simulink model "ScpAp_L1SpeedMonitor"  (R2025b)
settings: Solver=FixedStepDiscrete  StartTime=0.0  StopTime=10.0  FixedStep=0.01  RelTol=1e-3
model workspace (MAT data in the model file):
  Accel_Max = Simulink.Parameter
  Accel_Max.Value = 32.767
  Accel_Max.Complexity = 'real'
  Accel_Max.Dimensions = [1 1]
  Accel_Max.DataType = 'double'
  Alpha_Accel_IMU = Simulink.Parameter
  Alpha_Accel_IMU.Value = 0.15
  Alpha_Accel_IMU.Complexity = 'real'
  Alpha_Accel_IMU.Dimensions = [1 1]
  Alpha_Accel_IMU.DataType = 'double'
  Alpha_Motor = Simulink.Parameter
  Alpha_Motor.Value = 0.45
  Alpha_Motor.Complexity = 'real'
  Alpha_Motor.Dimensions = [1 1]
  Alpha_Motor.DataType = 'double'
  Alpha_WSS = Simulink.Parameter
  Alpha_WSS.Value = 0.35
  Alpha_WSS.Complexity = 'real'
  Alpha_WSS.Dimensions = [1 1]
  Alpha_WSS.DataType = 'double'
  Motor_Spd_Max = Simulink.Parameter
  Motor_Spd_Max.Value = 1023
  Motor_Spd_Max.Complexity = 'real'
  Motor_Spd_Max.Dimensions = [1 1]
  Motor_Spd_Max.DataType = 'uint16'
  Motor_Spd_Min = Simulink.Parameter
  Motor_Spd_Min.Value = 0
  Motor_Spd_Min.Complexity = 'real'
  Motor_Spd_Min.Dimensions = [1 1]
  Motor_Spd_Min.DataType = 'uint16'
  WhlSpd_Max = Simulink.Parameter
  WhlSpd_Max.Value = 32
  WhlSpd_Max.Complexity = 'real'
  WhlSpd_Max.Dimensions = [1 1]
  WhlSpd_Max.DataType = 'uint16'
  WhlSpd_Min = Simulink.Parameter
  WhlSpd_Min.Value = 0
  WhlSpd_Min.Complexity = 'real'
  WhlSpd_Min.Dimensions = [1 1]
  WhlSpd_Min.DataType = 'uint16'
undefined symbols (not defined in the file): IMU_Stuck_Delta, Motor_Stuck_Delta, Stuck_Th_Cyc, Wheel_Spd_Th, Whl_Stuck_Delta, WSS_Avg_Spd
settings Model: DataDictionary=EgasPOC.sldd  Creator=IAST283  LastModifiedBy=IAST283
settings DataIOCC: SaveFormat=StructureWithTime
settings OptimizationCC: DefaultParameterBehavior=Inlined  EnhancedBackFolding=on  PassReuseOutputArgsAs=Individual arguments  ZeroExternalMemoryAtStartup=off  ZeroInternalMemoryAtStartup=off  OptimizeBlockOrder=speed  DifferentSizesBufferReuse=on  OptimizationCustomize=off  EfficientTunableParamExpr=on
settings DebuggingCC: ParameterPrecisionLossMsg=none  ParameterTunabilityLossMsg=error
settings SFSimCC: MATLABDynamicMemAlloc=off
settings RTWCC: SystemTargetFile=autosar.tlc  GenCodeOnly=on  TemplateMakefile=ert_default_tmf  GenerateReport=on  DataTypeReplacement=CDataTypesFixedWidth  Description=AUTOSAR
settings CodeAppCC: ForceParamTrailComments=on  IgnoreCustomStorageClasses=off  OperatorAnnotations=on  SimulinkDataObjDesc=on  SFDataObjDesc=on  InsertBlockDesc=on
settings STFCustomTargetCC: SystemTargetFile=autosar.tlc  TargetLangStandard=C99 (ISO)  MultiwordLength=256.0  ParMdlRefBuildCompliant=on  CompOptLevelCompliant=on  ConcurrentExecutionCompliant=off  IncludeMdlTerminateFcn=off  CombineOutputUpdateFcns=on  SuppressErrorStatus=on  ERTCustomFileBanners=on  SupportNonFinite=off  SupportComplex=off  SupportContinuousTime=off  SupportNonInlinedSFcns=off  RemoveResetFunc=on  MATLABClassNameForMDSCustomization=Simulink.SoftwareTarget.ERTCustomization  AutosarCompliant=on  GRTInterface=off  UseToolchainInfoCompliant=on  LookupTableObjectStructAxisOrder=2,1,3,4,...  LUTObjectStructOrderEvenSpacing=Size,Table,Breakpoints  AutosarMatrixIOAsArray=off  DisableAUTOSARRoutinesHostLibrary=off  AutosarCompilerAbstraction=off  AutosarSchemaVersion=R23-11  AutosarMaxShortNameLength=128.0
settings ERTTargetCC: ERTCustomFileTemplate=example_file_process.tlc  BooleanTrueId=TRUE  BooleanFalseId=FALSE  TargetLangStandard=C99 (ISO)  ConcurrentExecutionCompliant=off  IncludeMdlTerminateFcn=off  SuppressErrorStatus=on  SupportNonFinite=off  SupportComplex=off  ModelStepFunctionPrototypeControlCompliant=off  CPPClassGenCompliant=off  AutosarCompliant=on  LookupTableObjectStructAxisOrder=2,1,3,4,...  LUTObjectStructOrderEvenSpacing=Size,Table,Breakpoints

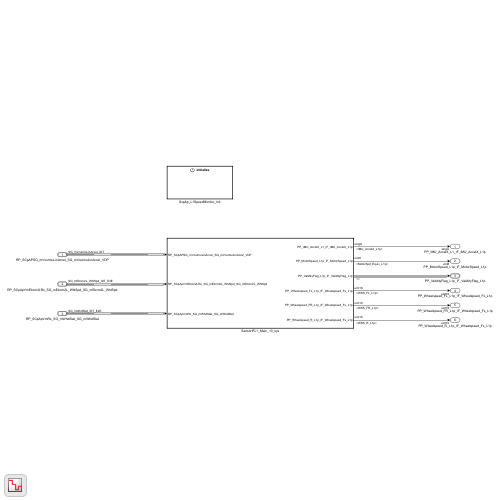
[thumbnail: Simulink's stored preview of the top-level diagram]
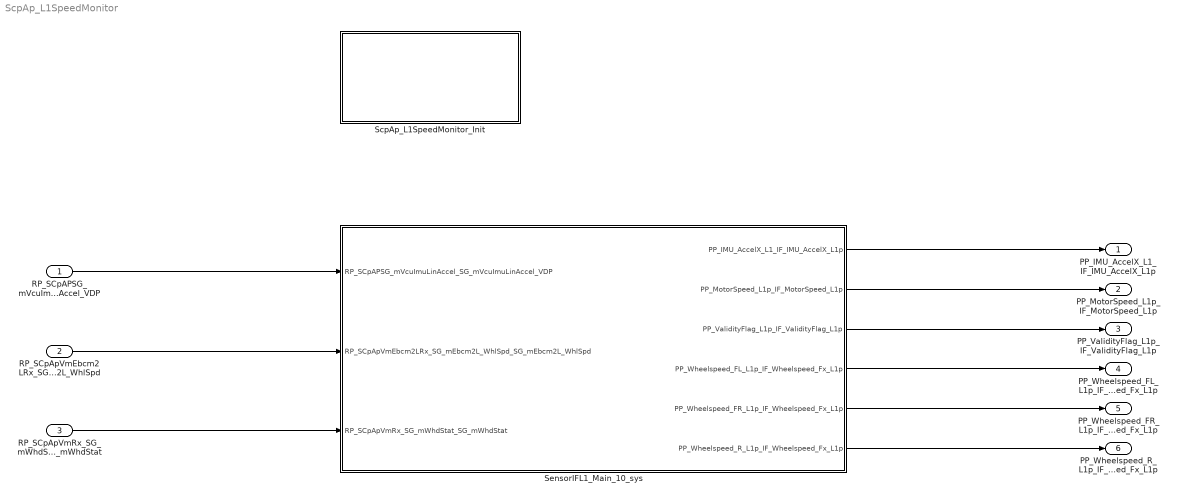
== system ScpAp_L1SpeedMonitor ==
  RP_SCpAPSG_mVcuImuLinAccel_SG_mVcuImuLinAccel_VDP : Inport  OutDataTypeStr=Bus: SG_mVcuImuLinAccel_IDT  PortDimensions=1  BusOutputAsStruct=on
  RP_SCpApVmEbcm2LRx_SG_mEbcm2L_WhlSpd_SG_mEbcm2L_WhlSpd : Inport  Port=2  OutDataTypeStr=Bus: SG_mEbcm2L_WhlSpd_IDT_E2E  PortDimensions=1  BusOutputAsStruct=on
  RP_SCpApVmRx_SG_mWhdStat_SG_mWhdStat : Inport  Port=3  OutDataTypeStr=Bus: SG_mWhdStat_IDT_E2E  PortDimensions=1  BusOutputAsStruct=on
  ScpAp_L1SpeedMonitor_Init : Subsystem
  SensorIFL1_Main_10_sys : Subsystem  TreatAsAtomicUnit=on  SystemSampleTime=0.01
  PP_IMU_AccelX_L1_IF_IMU_AccelX_L1p : Outport  OutDataTypeStr=single  PortDimensions=1
  PP_MotorSpeed_L1p_IF_MotorSpeed_L1p : Outport  Port=2  OutDataTypeStr=uint8  PortDimensions=1
  PP_ValidityFlag_L1p_IF_ValidityFlag_L1p : Outport  Port=3  OutDataTypeStr=Bus: IF_ValidityFlag_L1p_IDT  PortDimensions=1  BusOutputAsStruct=on
  PP_Wheelspeed_FL_L1p_IF_Wheelspeed_Fx_L1p : Outport  Port=4  OutDataTypeStr=uint16  PortDimensions=1
  PP_Wheelspeed_FR_L1p_IF_Wheelspeed_Fx_L1p : Outport  Port=5  OutDataTypeStr=uint16  PortDimensions=1
  PP_Wheelspeed_R_L1p_IF_Wheelspeed_Fx_L1p : Outport  Port=6  OutDataTypeStr=uint16  PortDimensions=1
  wires:
  RP_SCpAPSG_mVcuImuLinAccel_SG_mVcuImuLinAccel_VDP/1 -> SensorIFL1_Main_10_sys/1(RP_SCpAPSG_mVcuImuLinAccel_SG_mVcuImuLinAccel_VDP)
  RP_SCpApVmEbcm2LRx_SG_mEbcm2L_WhlSpd_SG_mEbcm2L_WhlSpd/1 -> SensorIFL1_Main_10_sys/2(RP_SCpApVmEbcm2LRx_SG_mEbcm2L_WhlSpd_SG_mEbcm2L_WhlSpd)
  RP_SCpApVmRx_SG_mWhdStat_SG_mWhdStat/1 -> SensorIFL1_Main_10_sys/3(RP_SCpApVmRx_SG_mWhdStat_SG_mWhdStat)
  SensorIFL1_Main_10_sys/1(PP_IMU_AccelX_L1_IF_IMU_AccelX_L1p) -> PP_IMU_AccelX_L1_IF_IMU_AccelX_L1p/1
  SensorIFL1_Main_10_sys/2(PP_MotorSpeed_L1p_IF_MotorSpeed_L1p) -> PP_MotorSpeed_L1p_IF_MotorSpeed_L1p/1
  SensorIFL1_Main_10_sys/3(PP_ValidityFlag_L1p_IF_ValidityFlag_L1p) -> PP_ValidityFlag_L1p_IF_ValidityFlag_L1p/1
  SensorIFL1_Main_10_sys/4(PP_Wheelspeed_FL_L1p_IF_Wheelspeed_Fx_L1p) -> PP_Wheelspeed_FL_L1p_IF_Wheelspeed_Fx_L1p/1
  SensorIFL1_Main_10_sys/5(PP_Wheelspeed_FR_L1p_IF_Wheelspeed_Fx_L1p) -> PP_Wheelspeed_FR_L1p_IF_Wheelspeed_Fx_L1p/1
  SensorIFL1_Main_10_sys/6(PP_Wheelspeed_R_L1p_IF_Wheelspeed_Fx_L1p) -> PP_Wheelspeed_R_L1p_IF_Wheelspeed_Fx_L1p/1

== system ScpAp_L1SpeedMonitor/ScpAp_L1SpeedMonitor_Init ==
  Event Listener : EventListener  EventName=reset

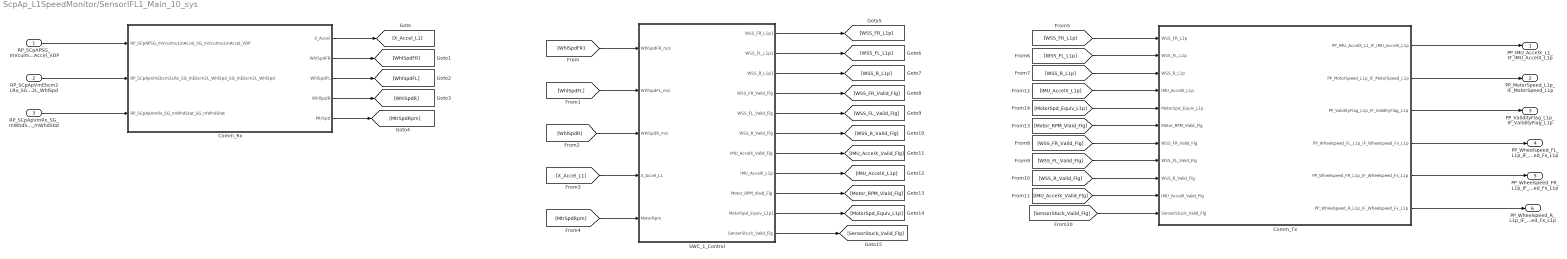
== system ScpAp_L1SpeedMonitor/SensorIFL1_Main_10_sys ==
  RP_SCpAPSG_mVcuImuLinAccel_SG_mVcuImuLinAccel_VDP : Inport
  RP_SCpApVmEbcm2LRx_SG_mEbcm2L_WhlSpd_SG_mEbcm2L_WhlSpd : Inport  Port=2
  RP_SCpApVmRx_SG_mWhdStat_SG_mWhdStat : Inport  Port=3
  Comm_Rx : Subsystem
  Comm_Tx : Subsystem
  SWC_1_Control : Subsystem  TreatAsAtomicUnit=on
  PP_IMU_AccelX_L1_IF_IMU_AccelX_L1p : Outport
  PP_MotorSpeed_L1p_IF_MotorSpeed_L1p : Outport  Port=2
  PP_ValidityFlag_L1p_IF_ValidityFlag_L1p : Outport  Port=3
  PP_Wheelspeed_FL_L1p_IF_Wheelspeed_Fx_L1p : Outport  Port=4
  PP_Wheelspeed_FR_L1p_IF_Wheelspeed_Fx_L1p : Outport  Port=5
  PP_Wheelspeed_R_L1p_IF_Wheelspeed_Fx_L1p : Outport  Port=6
  wires:
  Comm_Rx/3(WhlSpdFL) -> [WhlSpdFL]
  Comm_Rx/5(MtrSpd) -> [MtrSpdRpm]
  Comm_Rx/4(WhlSpdR) -> [WhlSpdR]
  Comm_Rx/2(WhlSpdFR) -> [WhlSpdFR]
  Comm_Rx/1(X_Accel) -> [X_Accel_L1]
  RP_SCpAPSG_mVcuImuLinAccel_SG_mVcuImuLinAccel_VDP/1 -> Comm_Rx/1(RP_SCpAPSG_mVcuImuLinAccel_SG_mVcuImuLinAccel_VDP)
  RP_SCpApVmRx_SG_mWhdStat_SG_mWhdStat/1 -> Comm_Rx/3(RP_SCpApVmRx_SG_mWhdStat_SG_mWhdStat)
  RP_SCpApVmEbcm2LRx_SG_mEbcm2L_WhlSpd_SG_mEbcm2L_WhlSpd/1 -> Comm_Rx/2(RP_SCpApVmEbcm2LRx_SG_mEbcm2L_WhlSpd_SG_mEbcm2L_WhlSpd)
  SWC_1_Control/7(IMU_AccelX_Valid_Flg) -> [IMU_AccelX_Valid_Flg]
  [WhlSpdFL] -> SWC_1_Control/2(WhlSpdFL_m/s)
  SWC_1_Control/1(WSS_FR_L1p1) -> [WSS_FR_L1p]
  SWC_1_Control/4(WSS_FR_Valid_Flg) -> [WSS_FR_Valid_Flg]
  SWC_1_Control/6(WSS_R_Valid_Flg) -> [WSS_R_Valid_Flg]
  SWC_1_Control/2(WSS_FL_L1p1) -> [WSS_FL_L1p]
  SWC_1_Control/11(SensorStuck_Valid_Flg) -> [SensorStuck_Valid_Flg]
  SWC_1_Control/9(Motor_RPM_Vlaid_Flg) -> [Motor_RPM_Vlaid_Flg]
  SWC_1_Control/10(MotorSpd_Equiv_L1p1) -> [MotorSpd_Equiv_L1p]
  SWC_1_Control/8(IMU_AccelX_L1p) -> [IMU_AccelX_L1p]
  SWC_1_Control/3(WSS_R_L1p1) -> [WSS_R_L1p]
  [MtrSpdRpm] -> SWC_1_Control/5(MotorRpm)
  [WhlSpdFR] -> SWC_1_Control/1(WhlSpdFR_m/s)
  [WhlSpdR] -> SWC_1_Control/3(WhlSpdR_m/s)
  SWC_1_Control/5(WSS_FL_Valid_Flg) -> [WSS_FL_Valid_Flg]
  [X_Accel_L1] -> SWC_1_Control/4(X_Accel_L1)
  [WSS_FR_L1p] -> Comm_Tx/1(WSS_FR_L1p)
  [WSS_FL_L1p] -> Comm_Tx/2(WSS_FL_L1p)
  [WSS_R_L1p] -> Comm_Tx/3(WSS_R_L1p)
  [IMU_AccelX_L1p] -> Comm_Tx/4(IMU_AccelX_L1p)
  [MotorSpd_Equiv_L1p] -> Comm_Tx/5(MotorSpd_Equiv_L1p)
  [Motor_RPM_Vlaid_Flg] -> Comm_Tx/6(Motor_RPM_Valid_Flg)
  [WSS_FR_Valid_Flg] -> Comm_Tx/7(WSS_FR_Valid_Flg)
  [WSS_FL_Valid_Flg] -> Comm_Tx/8(WSS_FL_Valid_Flg)
  [SensorStuck_Valid_Flg] -> Comm_Tx/11(SensorStuck_Valid_Flg)
  [IMU_AccelX_Valid_Flg] -> Comm_Tx/10(IMU_AccelX_Valid_Flg)
  [WSS_R_Valid_Flg] -> Comm_Tx/9(WSS_R_Valid_Flg)
  Comm_Tx/1(PP_IMU_AccelX_L1_IF_IMU_AccelX_L1p) -> PP_IMU_AccelX_L1_IF_IMU_AccelX_L1p/1
  Comm_Tx/2(PP_MotorSpeed_L1p_IF_MotorSpeed_L1p) -> PP_MotorSpeed_L1p_IF_MotorSpeed_L1p/1
  Comm_Tx/3(PP_ValidityFlag_L1p_IF_ValidityFlag_L1p) -> PP_ValidityFlag_L1p_IF_ValidityFlag_L1p/1
  Comm_Tx/4(PP_Wheelspeed_FL_L1p_IF_Wheelspeed_Fx_L1p) -> PP_Wheelspeed_FL_L1p_IF_Wheelspeed_Fx_L1p/1
  Comm_Tx/5(PP_Wheelspeed_FR_L1p_IF_Wheelspeed_Fx_L1p) -> PP_Wheelspeed_FR_L1p_IF_Wheelspeed_Fx_L1p/1
  Comm_Tx/6(PP_Wheelspeed_R_L1p_IF_Wheelspeed_Fx_L1p) -> PP_Wheelspeed_R_L1p_IF_Wheelspeed_Fx_L1p/1

== system ScpAp_L1SpeedMonitor/SensorIFL1_Main_10_sys/Comm_Rx ==
  RP_SCpAPSG_mVcuImuLinAccel_SG_mVcuImuLinAccel_VDP : Inport
  RP_SCpApVmEbcm2LRx_SG_mEbcm2L_WhlSpd_SG_mEbcm2L_WhlSpd : Inport  Port=2
  RP_SCpApVmRx_SG_mWhdStat_SG_mWhdStat : Inport  Port=3
  mEbcm2L_WhlSpd : Subsystem
  mVculmuLinAccel : Subsystem
  mWhdStat : Subsystem
  X_Accel : Outport
  WhlSpdFR : Outport  Port=2
  WhlSpdFL : Outport  Port=3
  WhlSpdR : Outport  Port=4
  MtrSpd : Outport  Port=5
  wires:
  mEbcm2L_WhlSpd/1(WhlSpdFR) -> WhlSpdFR/1
  mEbcm2L_WhlSpd/2(WhlSpdFL) -> WhlSpdFL/1
  mEbcm2L_WhlSpd/3(WhlSpdR) -> WhlSpdR/1
  RP_SCpApVmEbcm2LRx_SG_mEbcm2L_WhlSpd_SG_mEbcm2L_WhlSpd/1 -> mEbcm2L_WhlSpd/1(RP_SCpApVmEbcm2LRx_SG_mEbcm2L_WhlSpd_SG_mEbcm2L_WhlSpd)
  RP_SCpAPSG_mVcuImuLinAccel_SG_mVcuImuLinAccel_VDP/1 -> mVculmuLinAccel/1(RP_SCpAPSG_mVcuImuLinAccel_SG_mVcuImuLinAccel_VDP)
  RP_SCpApVmRx_SG_mWhdStat_SG_mWhdStat/1 -> mWhdStat/1(RP_SCpApVmRx_SG_mWhdStat_SG_mWhdStat)
  mWhdStat/1(MtrSpd) -> MtrSpd/1
  mVculmuLinAccel/1(X_Accel) -> X_Accel/1

== system ScpAp_L1SpeedMonitor/SensorIFL1_Main_10_sys/Comm_Tx ==
  WSS_FR_L1p : Inport
  WSS_FL_L1p : Inport  Port=2
  WSS_R_L1p : Inport  Port=3
  IMU_AccelX_L1p : Inport  Port=4
  MotorSpd_Equiv_L1p : Inport  Port=5
  Motor_RPM_Valid_Flg : Inport  Port=6
  WSS_FR_Valid_Flg : Inport  Port=7
  WSS_FL_Valid_Flg : Inport  Port=8
  WSS_R_Valid_Flg : Inport  Port=9
  IMU_AccelX_Valid_Flg : Inport  Port=10
  SensorStuck_Valid_Flg : Inport  Port=11
  Bus Creator : BusCreator  Inputs=6
  PP_IMU_AccelX_L1_IF_IMU_AccelX_L1p : Outport
  PP_MotorSpeed_L1p_IF_MotorSpeed_L1p : Outport  Port=2
  PP_ValidityFlag_L1p_IF_ValidityFlag_L1p : Outport  Port=3
  PP_Wheelspeed_FL_L1p_IF_Wheelspeed_Fx_L1p : Outport  Port=4
  PP_Wheelspeed_FR_L1p_IF_Wheelspeed_Fx_L1p : Outport  Port=5
  PP_Wheelspeed_R_L1p_IF_Wheelspeed_Fx_L1p : Outport  Port=6
  wires:
  WSS_FL_L1p/1 -> PP_Wheelspeed_FL_L1p_IF_Wheelspeed_Fx_L1p/1  "WSS_FL_L1p"
  WSS_FR_L1p/1 -> PP_Wheelspeed_FR_L1p_IF_Wheelspeed_Fx_L1p/1  "WSS_FR_L1p"
  WSS_R_L1p/1 -> PP_Wheelspeed_R_L1p_IF_Wheelspeed_Fx_L1p/1  "WSS_R_L1p"
  IMU_AccelX_L1p/1 -> PP_IMU_AccelX_L1_IF_IMU_AccelX_L1p/1  "IMU_AccelX_L1p"
  MotorSpd_Equiv_L1p/1 -> PP_MotorSpeed_L1p_IF_MotorSpeed_L1p/1  "MotorSpd_Equiv_L1p"
  Bus Creator/1 -> PP_ValidityFlag_L1p_IF_ValidityFlag_L1p/1
  Motor_RPM_Valid_Flg/1 -> Bus Creator/1
  WSS_FR_Valid_Flg/1 -> Bus Creator/2
  WSS_FL_Valid_Flg/1 -> Bus Creator/3
  WSS_R_Valid_Flg/1 -> Bus Creator/4
  IMU_AccelX_Valid_Flg/1 -> Bus Creator/5
  SensorStuck_Valid_Flg/1 -> Bus Creator/6

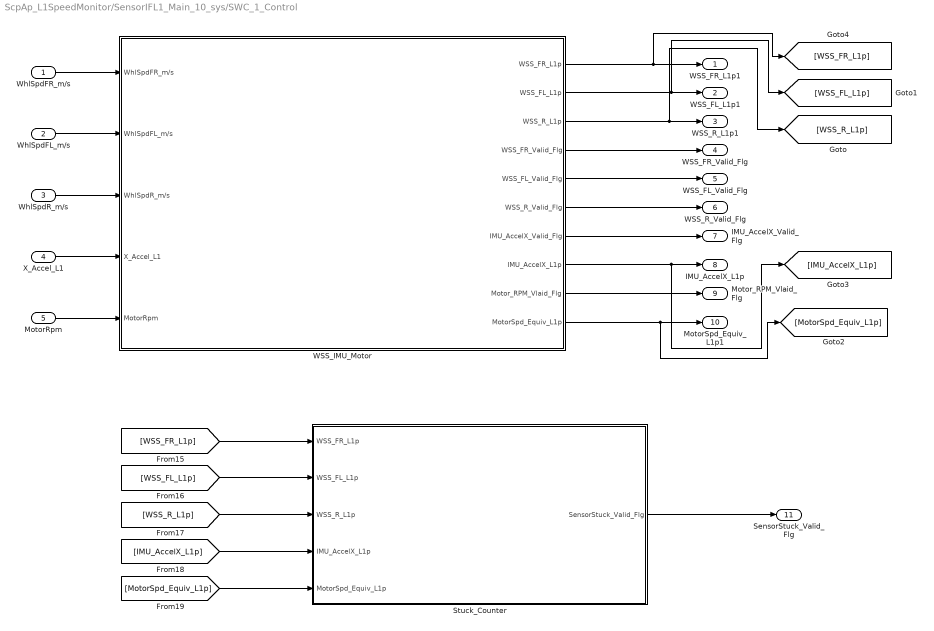
== system ScpAp_L1SpeedMonitor/SensorIFL1_Main_10_sys/SWC_1_Control ==
  WhlSpdFR_m/s : Inport
  WhlSpdFL_m/s : Inport  Port=2
  WhlSpdR_m/s : Inport  Port=3
  X_Accel_L1 : Inport  Port=4
  MotorRpm : Inport  Port=5
  Stuck_Counter : Subsystem  TreatAsAtomicUnit=on
  WSS_IMU_Motor : Subsystem  TreatAsAtomicUnit=on
  WSS_FR_L1p1 : Outport
  WSS_FL_L1p1 : Outport  Port=2
  WSS_R_L1p1 : Outport  Port=3
  WSS_FR_Valid_Flg : Outport  Port=4
  WSS_FL_Valid_Flg : Outport  Port=5
  WSS_R_Valid_Flg : Outport  Port=6
  IMU_AccelX_Valid_Flg : Outport  Port=7
  IMU_AccelX_L1p : Outport  Port=8
  Motor_RPM_Vlaid_Flg : Outport  Port=9
  MotorSpd_Equiv_L1p1 : Outport  Port=10
  SensorStuck_Valid_Flg : Outport  Port=11
  wires:
  WSS_IMU_Motor/6(WSS_R_Valid_Flg) -> WSS_R_Valid_Flg/1
  WSS_IMU_Motor/1(WSS_FR_L1p) -> WSS_FR_L1p1/1, [WSS_FR_L1p]
  WSS_IMU_Motor/9(Motor_RPM_Vlaid_Flg) -> Motor_RPM_Vlaid_Flg/1
  WSS_IMU_Motor/2(WSS_FL_L1p) -> [WSS_FL_L1p], WSS_FL_L1p1/1
  WSS_IMU_Motor/4(WSS_FR_Valid_Flg) -> WSS_FR_Valid_Flg/1
  WSS_IMU_Motor/8(IMU_AccelX_L1p) -> [IMU_AccelX_L1p], IMU_AccelX_L1p/1
  WSS_IMU_Motor/7(IMU_AccelX_Valid_Flg) -> IMU_AccelX_Valid_Flg/1
  X_Accel_L1/1 -> WSS_IMU_Motor/4(X_Accel_L1)
  Stuck_Counter/1(SensorStuck_Valid_Flg) -> SensorStuck_Valid_Flg/1
  WhlSpdR_m/s/1 -> WSS_IMU_Motor/3(WhlSpdR_m/s)
  WhlSpdFR_m/s/1 -> WSS_IMU_Motor/1(WhlSpdFR_m/s)
  WSS_IMU_Motor/3(WSS_R_L1p) -> [WSS_R_L1p], WSS_R_L1p1/1
  MotorRpm/1 -> WSS_IMU_Motor/5(MotorRpm)
  WSS_IMU_Motor/10(MotorSpd_Equiv_L1p) -> [MotorSpd_Equiv_L1p], MotorSpd_Equiv_L1p1/1
  WSS_IMU_Motor/5(WSS_FL_Valid_Flg) -> WSS_FL_Valid_Flg/1
  WhlSpdFL_m/s/1 -> WSS_IMU_Motor/2(WhlSpdFL_m/s)
  [WSS_FR_L1p] -> Stuck_Counter/1(WSS_FR_L1p)
  [WSS_FL_L1p] -> Stuck_Counter/2(WSS_FL_L1p)
  [WSS_R_L1p] -> Stuck_Counter/3(WSS_R_L1p)
  [IMU_AccelX_L1p] -> Stuck_Counter/4(IMU_AccelX_L1p)
  [MotorSpd_Equiv_L1p] -> Stuck_Counter/5(MotorSpd_Equiv_L1p)

== system ScpAp_L1SpeedMonitor/SensorIFL1_Main_10_sys/Comm_Rx/mEbcm2L_WhlSpd ==
  RP_SCpApVmEbcm2LRx_SG_mEbcm2L_WhlSpd_SG_mEbcm2L_WhlSpd : Inport
  Bus Selector : BusSelector  OutputSignals=WhlSpdFR,WhlSpdFL,WhlSpdR
  WhlSpdFR : Outport
  WhlSpdFL : Outport  Port=2
  WhlSpdR : Outport  Port=3
  wires:
  RP_SCpApVmEbcm2LRx_SG_mEbcm2L_WhlSpd_SG_mEbcm2L_WhlSpd/1 -> Bus Selector/1
  Bus Selector/1 -> WhlSpdFR/1  "<WhlSpdFR>"
  Bus Selector/2 -> WhlSpdFL/1  "<WhlSpdFL>"
  Bus Selector/3 -> WhlSpdR/1  "<WhlSpdR>"

== system ScpAp_L1SpeedMonitor/SensorIFL1_Main_10_sys/Comm_Rx/mVculmuLinAccel ==
  RP_SCpAPSG_mVcuImuLinAccel_SG_mVcuImuLinAccel_VDP : Inport
  Bus Selector : BusSelector  OutputSignals=X_Accel
  X_Accel : Outport
  wires:
  RP_SCpAPSG_mVcuImuLinAccel_SG_mVcuImuLinAccel_VDP/1 -> Bus Selector/1
  Bus Selector/1 -> X_Accel/1  "<X_Accel>"

== system ScpAp_L1SpeedMonitor/SensorIFL1_Main_10_sys/Comm_Rx/mWhdStat ==
  RP_SCpApVmRx_SG_mWhdStat_SG_mWhdStat : Inport
  Bus Selector : BusSelector  OutputSignals=MtrSpd
  MtrSpd : Outport
  wires:
  RP_SCpApVmRx_SG_mWhdStat_SG_mWhdStat/1 -> Bus Selector/1
  Bus Selector/1 -> MtrSpd/1  "<MtrSpd>"

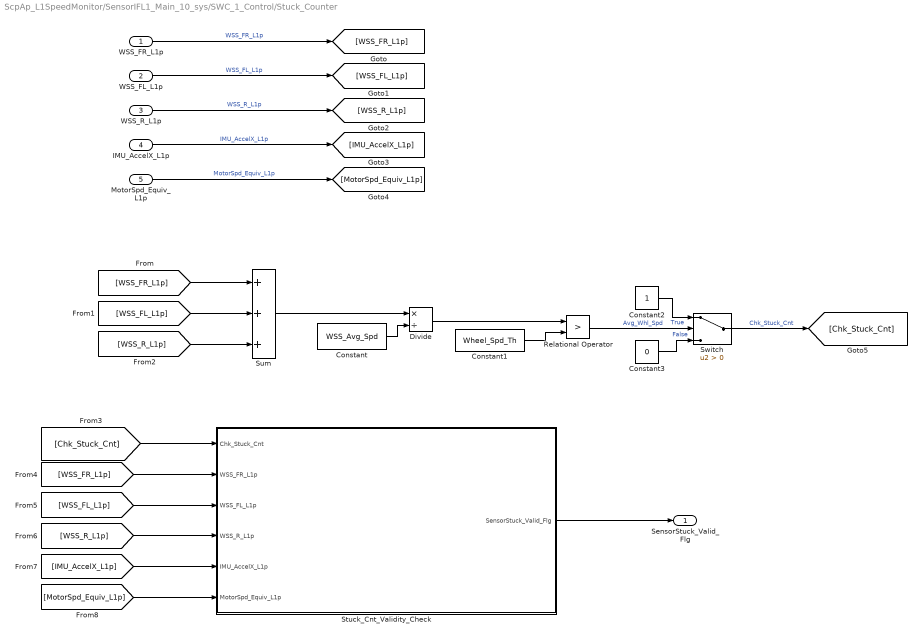
== system ScpAp_L1SpeedMonitor/SensorIFL1_Main_10_sys/SWC_1_Control/Stuck_Counter ==
  WSS_FR_L1p : Inport
  WSS_FL_L1p : Inport  Port=2
  WSS_R_L1p : Inport  Port=3
  IMU_AccelX_L1p : Inport  Port=4
  MotorSpd_Equiv_L1p : Inport  Port=5
  Constant : Constant  Value=WSS_Avg_Spd
  Constant1 : Constant  Value=Wheel_Spd_Th
  Constant2 : Constant  OutDataTypeStr=boolean
  Constant3 : Constant  Value=0  OutDataTypeStr=boolean
  Divide : Product  Inputs=*/
  Relational Operator : RelationalOperator  Operator=>  OutDataTypeStr=boolean  RndMeth=Simplest  InputSameDT=off
  Stuck_Cnt_Validity_Check : Subsystem  TreatAsAtomicUnit=on
  Sum : Sum  Inputs=+++
  Switch : Switch  Criteria=u2 > Threshold  SaturateOnIntegerOverflow=off  InputSameDT=off
  SensorStuck_Valid_Flg : Outport
  wires:
  WSS_FR_L1p/1 -> [WSS_FR_L1p]  "WSS_FR_L1p"
  WSS_FL_L1p/1 -> [WSS_FL_L1p]  "WSS_FL_L1p"
  WSS_R_L1p/1 -> [WSS_R_L1p]  "WSS_R_L1p"
  IMU_AccelX_L1p/1 -> [IMU_AccelX_L1p]  "IMU_AccelX_L1p"
  MotorSpd_Equiv_L1p/1 -> [MotorSpd_Equiv_L1p]  "MotorSpd_Equiv_L1p"
  [WSS_FR_L1p] -> Sum/1
  [WSS_FL_L1p] -> Sum/2
  [WSS_R_L1p] -> Sum/3
  Sum/1 -> Divide/1
  Constant/1 -> Divide/2
  Divide/1 -> Relational Operator/1
  Constant1/1 -> Relational Operator/2
  Relational Operator/1 -> Switch/2  "Avg_Whl_Spd"
  Constant2/1 -> Switch/1  "True"
  Constant3/1 -> Switch/3  "False"
  Switch/1 -> [Chk_Stuck_Cnt]  "Chk_Stuck_Cnt"
  [WSS_FR_L1p] -> Stuck_Cnt_Validity_Check/2(WSS_FR_L1p)
  [WSS_FL_L1p] -> Stuck_Cnt_Validity_Check/3(WSS_FL_L1p)
  [WSS_R_L1p] -> Stuck_Cnt_Validity_Check/4(WSS_R_L1p)
  [MotorSpd_Equiv_L1p] -> Stuck_Cnt_Validity_Check/6(MotorSpd_Equiv_L1p)
  [IMU_AccelX_L1p] -> Stuck_Cnt_Validity_Check/5(IMU_AccelX_L1p)
  [Chk_Stuck_Cnt] -> Stuck_Cnt_Validity_Check/1(Chk_Stuck_Cnt)
  Stuck_Cnt_Validity_Check/1(SensorStuck_Valid_Flg) -> SensorStuck_Valid_Flg/1

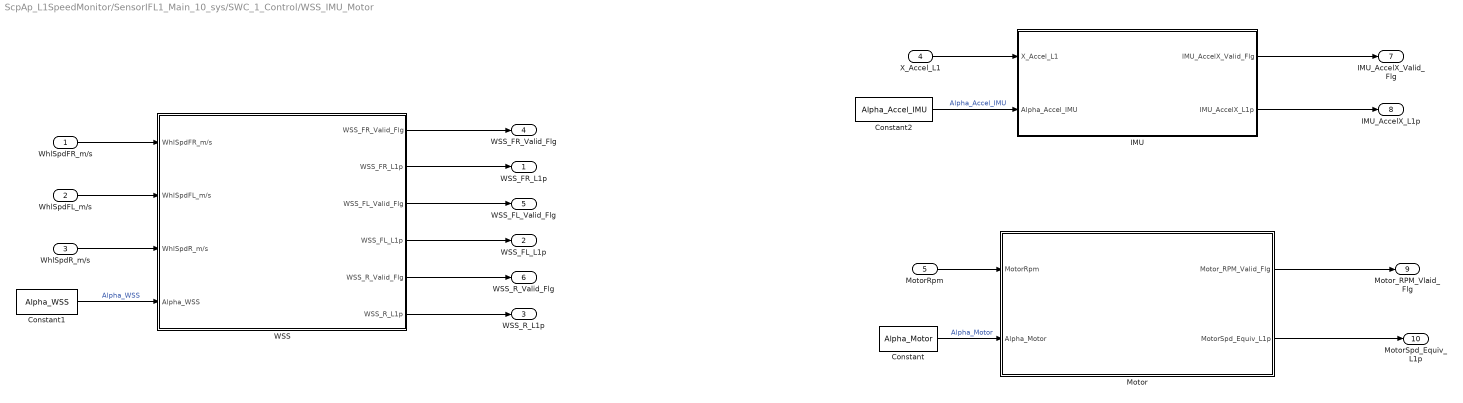
== system ScpAp_L1SpeedMonitor/SensorIFL1_Main_10_sys/SWC_1_Control/WSS_IMU_Motor ==
  WhlSpdFR_m/s : Inport
  WhlSpdFL_m/s : Inport  Port=2
  WhlSpdR_m/s : Inport  Port=3
  X_Accel_L1 : Inport  Port=4
  MotorRpm : Inport  Port=5
  Constant : Constant  Value=Alpha_Motor  OutDataTypeStr=double
  Constant1 : Constant  Value=Alpha_WSS  OutDataTypeStr=double
  Constant2 : Constant  Value=Alpha_Accel_IMU  OutDataTypeStr=double
  IMU : Subsystem  TreatAsAtomicUnit=on
  Motor : Subsystem  TreatAsAtomicUnit=on
  WSS : Subsystem  TreatAsAtomicUnit=on
  WSS_FR_L1p : Outport
  WSS_FL_L1p : Outport  Port=2
  WSS_R_L1p : Outport  Port=3
  WSS_FR_Valid_Flg : Outport  Port=4  OutDataTypeStr=boolean
  WSS_FL_Valid_Flg : Outport  Port=5
  WSS_R_Valid_Flg : Outport  Port=6
  IMU_AccelX_Valid_Flg : Outport  Port=7
  IMU_AccelX_L1p : Outport  Port=8
  Motor_RPM_Vlaid_Flg : Outport  Port=9
  MotorSpd_Equiv_L1p : Outport  Port=10
  wires:
  WSS/5(WSS_R_Valid_Flg) -> WSS_R_Valid_Flg/1
  WhlSpdR_m/s/1 -> WSS/3(WhlSpdR_m/s)
  WSS/3(WSS_FL_Valid_Flg) -> WSS_FL_Valid_Flg/1
  WSS/4(WSS_FL_L1p) -> WSS_FL_L1p/1
  WhlSpdFR_m/s/1 -> WSS/1(WhlSpdFR_m/s)
  WSS/1(WSS_FR_Valid_Flg) -> WSS_FR_Valid_Flg/1
  WSS/6(WSS_R_L1p) -> WSS_R_L1p/1
  WSS/2(WSS_FR_L1p) -> WSS_FR_L1p/1
  WhlSpdFL_m/s/1 -> WSS/2(WhlSpdFL_m/s)
  X_Accel_L1/1 -> IMU/1(X_Accel_L1)
  IMU/1(IMU_AccelX_Valid_Flg) -> IMU_AccelX_Valid_Flg/1
  IMU/2(IMU_AccelX_L1p) -> IMU_AccelX_L1p/1
  MotorRpm/1 -> Motor/1(MotorRpm)
  Motor/1(Motor_RPM_Valid_Flg) -> Motor_RPM_Vlaid_Flg/1
  Motor/2(MotorSpd_Equiv_L1p) -> MotorSpd_Equiv_L1p/1
  Constant/1 -> Motor/2(Alpha_Motor)  "Alpha_Motor"
  Constant1/1 -> WSS/4(Alpha_WSS)  "Alpha_WSS"
  Constant2/1 -> IMU/2(Alpha_Accel_IMU)  "Alpha_Accel_IMU"

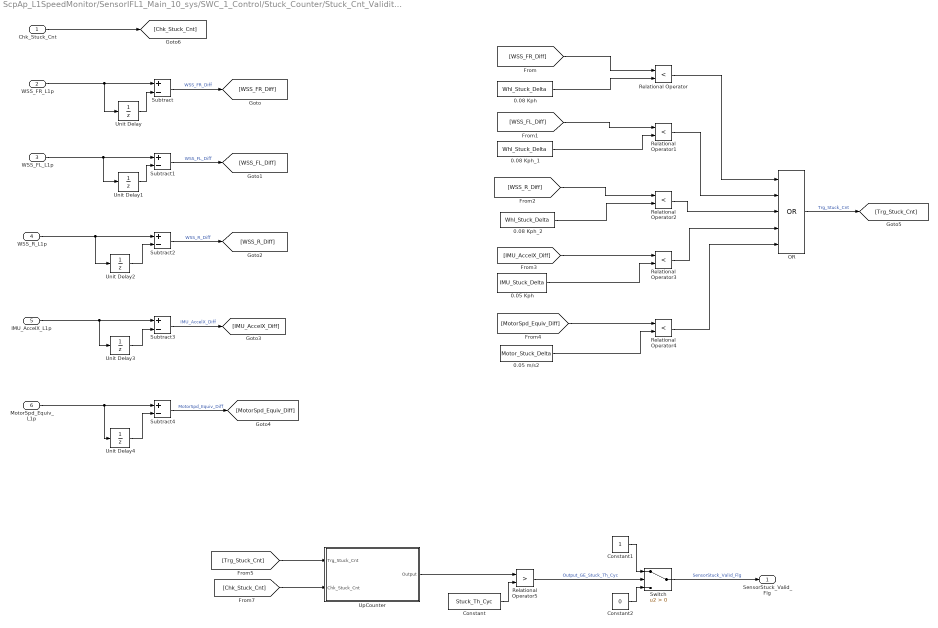
== system ScpAp_L1SpeedMonitor/SensorIFL1_Main_10_sys/SWC_1_Control/Stuck_Counter/Stuck_Cnt_Validity_Check ==
  Chk_Stuck_Cnt : Inport
  WSS_FR_L1p : Inport  Port=2
  WSS_FL_L1p : Inport  Port=3
  WSS_R_L1p : Inport  Port=4
  IMU_AccelX_L1p : Inport  Port=5
  MotorSpd_Equiv_L1p : Inport  Port=6
  0.05 Kph : Constant  Value=IMU_Stuck_Delta
  0.05 m/s2 : Constant  Value=Motor_Stuck_Delta
  0.08 Kph : Constant  Value=Whl_Stuck_Delta
  0.08 Kph_1 : Constant  Value=Whl_Stuck_Delta
  0.08 Kph_2 : Constant  Value=Whl_Stuck_Delta
  Constant : Constant  Value=Stuck_Th_Cyc
  Constant1 : Constant  OutDataTypeStr=boolean
  Constant2 : Constant  Value=0  OutDataTypeStr=boolean
  OR : Logic  Operator=OR  Inputs=5  IconShape=distinctive  AllPortsSameDT=off  OutDataTypeStr=boolean
  Relational Operator{,1..4} (5 alike) : RelationalOperator  Operator=<  OutDataTypeStr=boolean  RndMeth=Simplest  InputSameDT=off
  Relational Operator5 : RelationalOperator  Operator=>  OutDataTypeStr=boolean  RndMeth=Simplest  InputSameDT=off
  Subtract{,1..4} (5 alike) : Sum  Inputs=+-
  Switch : Switch  Criteria=u2 > Threshold  SaturateOnIntegerOverflow=off  InputSameDT=off
  Unit Delay{,1..4} (5 alike) : UnitDelay  SampleTime=-1  HasFrameUpgradeWarning=on
  UpCounter : Subsystem  TreatAsAtomicUnit=on
  SensorStuck_Valid_Flg : Outport
  wires:
  WSS_FR_L1p/1 -> Unit Delay/1, Subtract/1
  Subtract/1 -> [WSS_FR_Diff]  "WSS_FR_Diff"
  Unit Delay/1 -> Subtract/2
  WSS_FL_L1p/1 -> Unit Delay1/1, Subtract1/1
  Unit Delay1/1 -> Subtract1/2
  Subtract1/1 -> [WSS_FL_Diff]  "WSS_FL_Diff"
  WSS_R_L1p/1 -> Unit Delay2/1, Subtract2/1
  Unit Delay2/1 -> Subtract2/2
  Subtract2/1 -> [WSS_R_Diff]  "WSS_R_Diff"
  [WSS_FR_Diff] -> Relational Operator/1
  0.08 Kph/1 -> Relational Operator/2
  [WSS_FL_Diff] -> Relational Operator1/1
  0.08 Kph_1/1 -> Relational Operator1/2
  [WSS_R_Diff] -> Relational Operator2/1
  0.08 Kph_2/1 -> Relational Operator2/2
  IMU_AccelX_L1p/1 -> Unit Delay3/1, Subtract3/1
  Unit Delay3/1 -> Subtract3/2
  Subtract3/1 -> [IMU_AccelX_Diff]  "IMU_AccelX_Diff"
  MotorSpd_Equiv_L1p/1 -> Unit Delay4/1, Subtract4/1
  Subtract4/1 -> [MotorSpd_Equiv_Diff]  "MotorSpd_Equiv_Diff"
  Unit Delay4/1 -> Subtract4/2
  [IMU_AccelX_Diff] -> Relational Operator3/1
  0.05 Kph/1 -> Relational Operator3/2
  [MotorSpd_Equiv_Diff] -> Relational Operator4/1
  0.05 m/s2/1 -> Relational Operator4/2
  Relational Operator/1 -> OR/1
  Relational Operator1/1 -> OR/2
  Relational Operator2/1 -> OR/3
  Relational Operator3/1 -> OR/4
  Relational Operator4/1 -> OR/5
  OR/1 -> [Trg_Stuck_Cnt]  "Trg_Stuck_Cnt"
  Constant/1 -> Relational Operator5/2
  Relational Operator5/1 -> Switch/2  "Output_GE_Stuck_Th_Cyc"
  Constant1/1 -> Switch/1
  Constant2/1 -> Switch/3
  Switch/1 -> SensorStuck_Valid_Flg/1  "SensorStuck_Valid_Flg"
  Chk_Stuck_Cnt/1 -> [Chk_Stuck_Cnt]
  [Trg_Stuck_Cnt] -> UpCounter/1(Trg_Stuck_Cnt)
  [Chk_Stuck_Cnt] -> UpCounter/2(Chk_Stuck_Cnt)
  UpCounter/1(Output) -> Relational Operator5/1

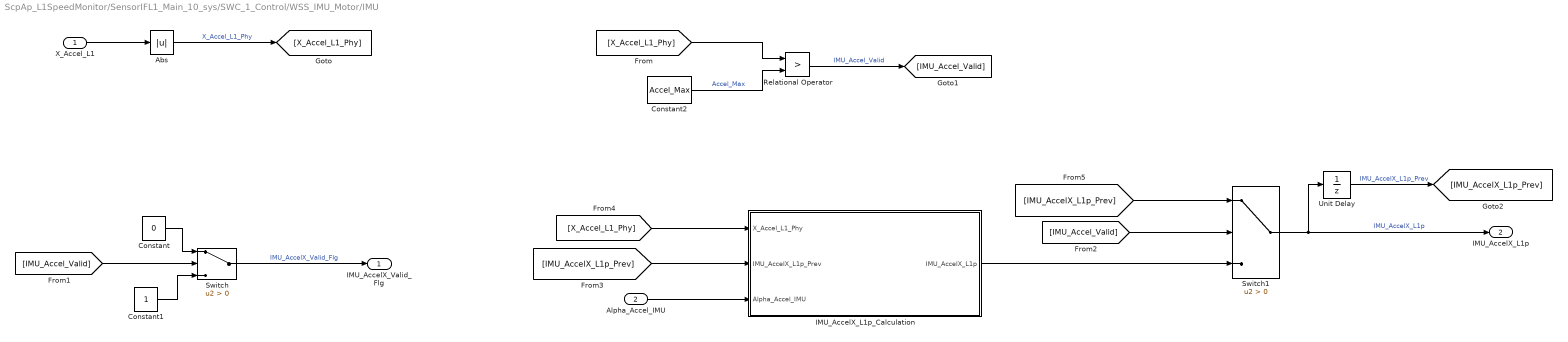
== system ScpAp_L1SpeedMonitor/SensorIFL1_Main_10_sys/SWC_1_Control/WSS_IMU_Motor/IMU ==
  X_Accel_L1 : Inport
  Alpha_Accel_IMU : Inport  Port=2
  Abs : Abs  SaturateOnIntegerOverflow=off
  Constant : Constant  Value=0  OutDataTypeStr=boolean
  Constant1 : Constant  OutDataTypeStr=boolean
  Constant2 : Constant  Value=Accel_Max
  IMU_AccelX_L1p_Calculation : Subsystem  TreatAsAtomicUnit=on
  Relational Operator : RelationalOperator  Operator=>  OutDataTypeStr=boolean  RndMeth=Simplest  InputSameDT=off
  Switch : Switch  Criteria=u2 > Threshold  SaturateOnIntegerOverflow=off  InputSameDT=off
  Switch1 : Switch  Criteria=u2 > Threshold  SaturateOnIntegerOverflow=off  InputSameDT=off
  Unit Delay : UnitDelay  SampleTime=-1  HasFrameUpgradeWarning=on
  IMU_AccelX_Valid_Flg : Outport
  IMU_AccelX_L1p : Outport  Port=2
  wires:
  Abs/1 -> [X_Accel_L1_Phy]  "X_Accel_L1_Phy"
  [X_Accel_L1_Phy] -> Relational Operator/1
  Constant2/1 -> Relational Operator/2  "Accel_Max"
  Relational Operator/1 -> [IMU_Accel_Valid]  "IMU_Accel_Valid"
  [IMU_Accel_Valid] -> Switch/2
  Constant/1 -> Switch/1
  Constant1/1 -> Switch/3
  Switch/1 -> IMU_AccelX_Valid_Flg/1  "IMU_AccelX_Valid_Flg"
  [IMU_Accel_Valid] -> Switch1/2
  Switch1/1 -> IMU_AccelX_L1p/1, Unit Delay/1  "IMU_AccelX_L1p"
  IMU_AccelX_L1p_Calculation/1(IMU_AccelX_L1p) -> Switch1/3
  Unit Delay/1 -> [IMU_AccelX_L1p_Prev]  "IMU_AccelX_L1p_Prev"
  [IMU_AccelX_L1p_Prev] -> IMU_AccelX_L1p_Calculation/2(IMU_AccelX_L1p_Prev)
  [X_Accel_L1_Phy] -> IMU_AccelX_L1p_Calculation/1(X_Accel_L1_Phy)
  [IMU_AccelX_L1p_Prev] -> Switch1/1
  Alpha_Accel_IMU/1 -> IMU_AccelX_L1p_Calculation/3(Alpha_Accel_IMU)
  X_Accel_L1/1 -> Abs/1

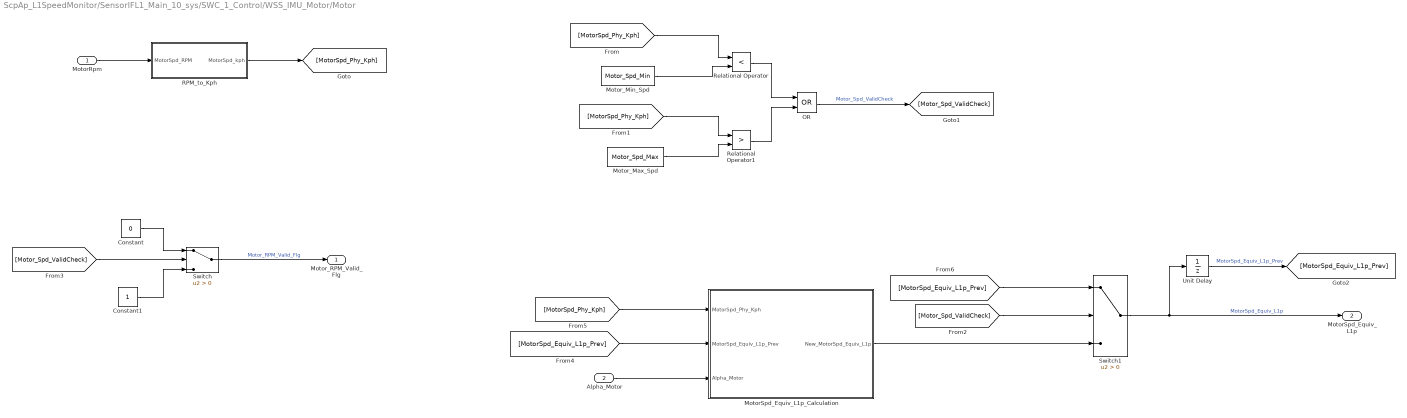
== system ScpAp_L1SpeedMonitor/SensorIFL1_Main_10_sys/SWC_1_Control/WSS_IMU_Motor/Motor ==
  MotorRpm : Inport
  Alpha_Motor : Inport  Port=2
  Constant : Constant  Value=0  OutDataTypeStr=boolean
  Constant1 : Constant  OutDataTypeStr=boolean
  MotorSpd_Equiv_L1p_Calculation : Subsystem  TreatAsAtomicUnit=on
  Motor_Max_Spd : Constant  Value=Motor_Spd_Max
  Motor_Min_Spd : Constant  Value=Motor_Spd_Min
  OR : Logic  Operator=OR  AllPortsSameDT=off  OutDataTypeStr=boolean
  RPM_to_Kph : Subsystem  TreatAsAtomicUnit=on
  Relational Operator : RelationalOperator  Operator=<  OutDataTypeStr=boolean  RndMeth=Simplest  InputSameDT=off
  Relational Operator1 : RelationalOperator  Operator=>  OutDataTypeStr=boolean  RndMeth=Simplest  InputSameDT=off
  Switch : Switch  Criteria=u2 > Threshold  SaturateOnIntegerOverflow=off  InputSameDT=off
  Switch1 : Switch  Criteria=u2 > Threshold  OutDataTypeStr=uint8  SaturateOnIntegerOverflow=off  InputSameDT=off
  Unit Delay : UnitDelay  SampleTime=-1  HasFrameUpgradeWarning=on
  Motor_RPM_Valid_Flg : Outport
  MotorSpd_Equiv_L1p : Outport  Port=2
  wires:
  RPM_to_Kph/1(MotorSpd_kph) -> [MotorSpd_Phy_Kph]
  [MotorSpd_Phy_Kph] -> Relational Operator/1
  Motor_Min_Spd/1 -> Relational Operator/2
  Relational Operator/1 -> OR/1
  [MotorSpd_Phy_Kph] -> Relational Operator1/1
  Motor_Max_Spd/1 -> Relational Operator1/2
  Relational Operator1/1 -> OR/2
  OR/1 -> [Motor_Spd_ValidCheck]  "Motor_Spd_ValidCheck"
  [Motor_Spd_ValidCheck] -> Switch/2
  Switch/1 -> Motor_RPM_Valid_Flg/1  "Motor_RPM_Valid_Flg"
  Constant/1 -> Switch/1
  Constant1/1 -> Switch/3
  [Motor_Spd_ValidCheck] -> Switch1/2
  Switch1/1 -> MotorSpd_Equiv_L1p/1, Unit Delay/1  "MotorSpd_Equiv_L1p"
  MotorSpd_Equiv_L1p_Calculation/1(New_MotorSpd_Equiv_L1p) -> Switch1/3
  Unit Delay/1 -> [MotorSpd_Equiv_L1p_Prev]  "MotorSpd_Equiv_L1p_Prev"
  [MotorSpd_Equiv_L1p_Prev] -> MotorSpd_Equiv_L1p_Calculation/2(MotorSpd_Equiv_L1p_Prev)
  [MotorSpd_Phy_Kph] -> MotorSpd_Equiv_L1p_Calculation/1(MotorSpd_Phy_Kph)
  Alpha_Motor/1 -> MotorSpd_Equiv_L1p_Calculation/3(Alpha_Motor)
  [MotorSpd_Equiv_L1p_Prev] -> Switch1/1
  MotorRpm/1 -> RPM_to_Kph/1(MotorSpd_RPM)

== system ScpAp_L1SpeedMonitor/SensorIFL1_Main_10_sys/SWC_1_Control/WSS_IMU_Motor/WSS ==
  WhlSpdFR_m/s : Inport
  WhlSpdFL_m/s : Inport  Port=2
  WhlSpdR_m/s : Inport  Port=3
  Alpha_WSS : Inport  Port=4  OutDataTypeStr=double
  WSS_FL : Subsystem  TreatAsAtomicUnit=on
  WSS_FR : Subsystem  TreatAsAtomicUnit=on
  WSS_R : Subsystem  TreatAsAtomicUnit=on
  WSS_FR_Valid_Flg : Outport  OutDataTypeStr=boolean
  WSS_FR_L1p : Outport  Port=2
  WSS_FL_Valid_Flg : Outport  Port=3
  WSS_FL_L1p : Outport  Port=4
  WSS_R_Valid_Flg : Outport  Port=5
  WSS_R_L1p : Outport  Port=6
  wires:
  Alpha_WSS/1 -> [Alpha_WSS]
  [Alpha_WSS] -> WSS_FR/2(Alpha_WSS)
  WSS_FR/1(WSS_FR_Valid_Flg) -> WSS_FR_Valid_Flg/1
  WSS_FR/2(WSS_FR_L1p) -> WSS_FR_L1p/1
  WhlSpdFL_m/s/1 -> WSS_FL/1(WhlSpdFL_m/s)
  [Alpha_WSS] -> WSS_FL/2(Alpha_WSS)
  WSS_FL/1(WSS_FL_Valid_Flg) -> WSS_FL_Valid_Flg/1
  WSS_FL/2(WSS_FL_L1p) -> WSS_FL_L1p/1
  WhlSpdR_m/s/1 -> WSS_R/1(WhlSpdR_m/s)
  [Alpha_WSS] -> WSS_R/2(Alpha_WSS)
  WSS_R/1(WSS_R_Valid_Flg) -> WSS_R_Valid_Flg/1
  WSS_R/2(WSS_R_L1p) -> WSS_R_L1p/1
  WhlSpdFR_m/s/1 -> WSS_FR/1(WhlSpdFR_m/s)

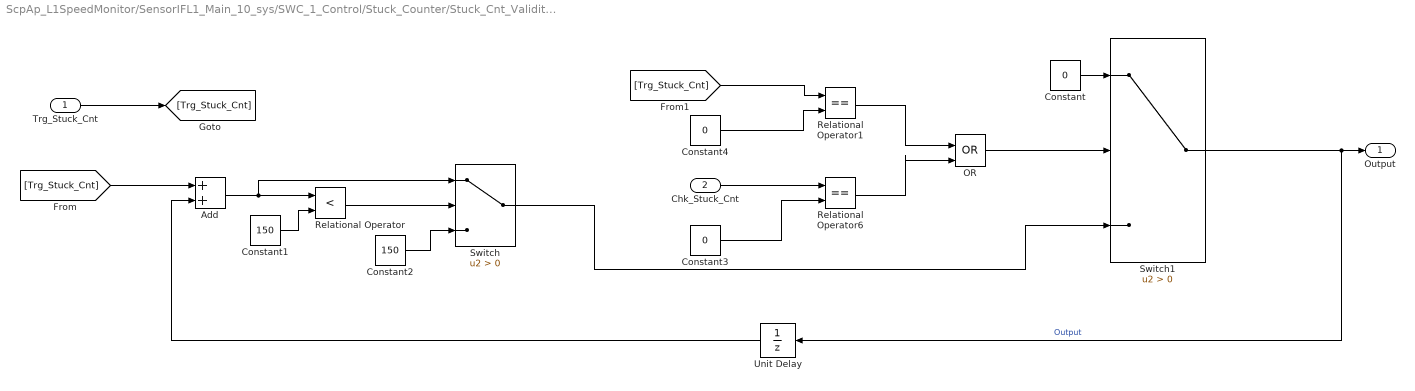
== system ScpAp_L1SpeedMonitor/SensorIFL1_Main_10_sys/SWC_1_Control/Stuck_Counter/Stuck_Cnt_Validity_Check/UpCounter ==
  Trg_Stuck_Cnt : Inport
  Chk_Stuck_Cnt : Inport  Port=2
  Add : Sum
  Constant : Constant  Value=0
  Constant1 : Constant  Value=150
  Constant2 : Constant  Value=150
  Constant3 : Constant  Value=0
  Constant4 : Constant  Value=0
  OR : Logic  Operator=OR  IconShape=distinctive  AllPortsSameDT=off  OutDataTypeStr=boolean
  Relational Operator : RelationalOperator  Operator=<  OutDataTypeStr=boolean  RndMeth=Simplest  InputSameDT=off
  Relational Operator1 : RelationalOperator  Operator===  OutDataTypeStr=boolean  RndMeth=Simplest  InputSameDT=off
  Relational Operator6 : RelationalOperator  Operator===  OutDataTypeStr=boolean  RndMeth=Simplest  InputSameDT=off
  Switch : Switch  Criteria=u2 > Threshold  SaturateOnIntegerOverflow=off  InputSameDT=off
  Switch1 : Switch  Criteria=u2 > Threshold  SaturateOnIntegerOverflow=off  InputSameDT=off
  Unit Delay : UnitDelay  SampleTime=-1  HasFrameUpgradeWarning=on
  Output : Outport
  wires:
  Constant2/1 -> Switch/3
  Unit Delay/1 -> Add/2
  Switch/1 -> Switch1/3
  Add/1 -> Relational Operator/1, Switch/1
  Constant1/1 -> Relational Operator/2
  Relational Operator/1 -> Switch/2
  Constant3/1 -> Relational Operator6/2
  Chk_Stuck_Cnt/1 -> Relational Operator6/1
  Constant/1 -> Switch1/1
  Switch1/1 -> Unit Delay/1, Output/1  "Output"
  Trg_Stuck_Cnt/1 -> [Trg_Stuck_Cnt]
  [Trg_Stuck_Cnt] -> Add/1
  Constant4/1 -> Relational Operator1/2
  [Trg_Stuck_Cnt] -> Relational Operator1/1
  OR/1 -> Switch1/2
  Relational Operator1/1 -> OR/1
  Relational Operator6/1 -> OR/2

== system ScpAp_L1SpeedMonitor/SensorIFL1_Main_10_sys/SWC_1_Control/WSS_IMU_Motor/IMU/IMU_AccelX_L1p_Calculation ==
  X_Accel_L1_Phy : Inport
  IMU_AccelX_L1p_Prev : Inport  Port=2
  Alpha_Accel_IMU : Inport  Port=3
  Add : Sum
  Constant : Constant  OutDataTypeStr=single
  Product : Product
  Product1 : Product
  Subtract : Sum  Inputs=+-
  IMU_AccelX_L1p : Outport
  wires:
  Alpha_Accel_IMU/1 -> [Alpha_Accel_IMU]
  [Alpha_Accel_IMU] -> Product/1
  X_Accel_L1_Phy/1 -> Product/2
  Constant/1 -> Subtract/1
  [Alpha_Accel_IMU] -> Subtract/2
  Subtract/1 -> Product1/1
  IMU_AccelX_L1p_Prev/1 -> Product1/2
  Product/1 -> Add/1
  Product1/1 -> Add/2
  Add/1 -> IMU_AccelX_L1p/1  "IMU_AccelX_L1p"

== system ScpAp_L1SpeedMonitor/SensorIFL1_Main_10_sys/SWC_1_Control/WSS_IMU_Motor/Motor/MotorSpd_Equiv_L1p_Calculation ==
  MotorSpd_Phy_Kph : Inport
  MotorSpd_Equiv_L1p_Prev : Inport  Port=2
  Alpha_Motor : Inport  Port=3
  Add : Sum
  Constant : Constant  OutDataTypeStr=uint8
  Product : Product  OutDataTypeStr=uint8
  Product1 : Product  OutDataTypeStr=uint8
  Subtract : Sum  Inputs=+-  OutDataTypeStr=uint8
  New_MotorSpd_Equiv_L1p : Outport
  wires:
  Alpha_Motor/1 -> [Alpha_Motor]
  [Alpha_Motor] -> Product/1
  MotorSpd_Phy_Kph/1 -> Product/2
  Constant/1 -> Subtract/1
  [Alpha_Motor] -> Subtract/2
  Subtract/1 -> Product1/1
  MotorSpd_Equiv_L1p_Prev/1 -> Product1/2
  Product/1 -> Add/1
  Product1/1 -> Add/2
  Add/1 -> New_MotorSpd_Equiv_L1p/1  "New_MotorSpd_Equiv_L1p"

== system ScpAp_L1SpeedMonitor/SensorIFL1_Main_10_sys/SWC_1_Control/WSS_IMU_Motor/Motor/RPM_to_Kph ==
  MotorSpd_RPM : Inport
  Constant : Constant  Value=2*pi
  Constant1 : Constant  Value=60
  Constant2 : Constant  Value=1000
  Data Type Conversion : DataTypeConversion  OutDataTypeStr=uint8  SaturateOnIntegerOverflow=off  RndMeth=Floor
  Divide : Product  Inputs=*/
  Product : Product  Inputs=4
  Radius_in_mm : Constant  Value=250
  MotorSpd_kph : Outport
  wires:
  MotorSpd_RPM/1 -> Product/3
  Constant/1 -> Product/1
  Radius_in_mm/1 -> Product/2
  Constant1/1 -> Product/4
  Product/1 -> Divide/1
  Constant2/1 -> Divide/2
  Divide/1 -> Data Type Conversion/1
  Data Type Conversion/1 -> MotorSpd_kph/1  "MotorSpd_kph"

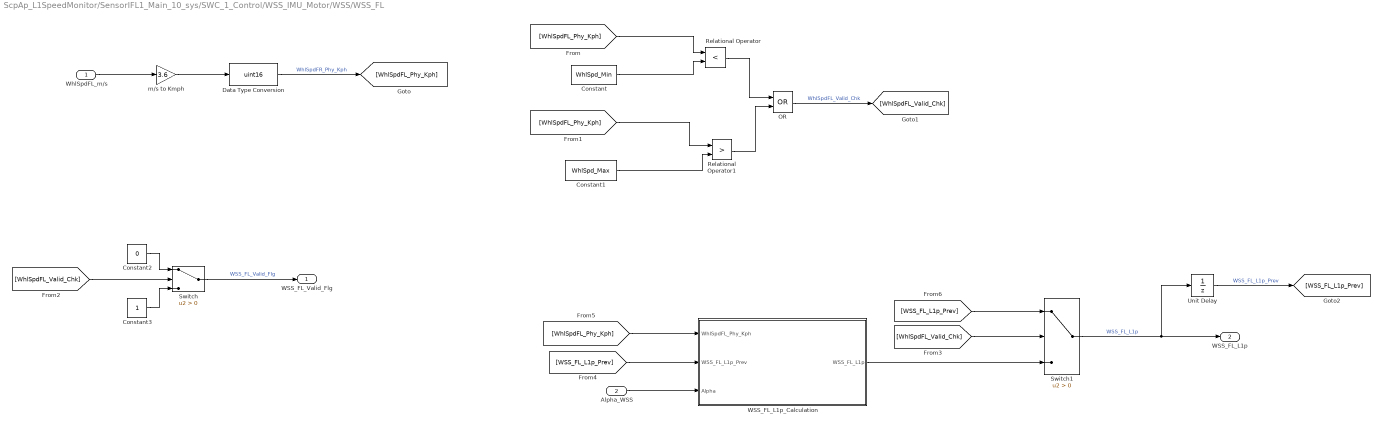
== system ScpAp_L1SpeedMonitor/SensorIFL1_Main_10_sys/SWC_1_Control/WSS_IMU_Motor/WSS/WSS_FL ==
  WhlSpdFL_m/s : Inport
  Alpha_WSS : Inport  Port=2
  Constant : Constant  Value=WhlSpd_Min
  Constant1 : Constant  Value=WhlSpd_Max
  Constant2 : Constant  Value=0  OutDataTypeStr=boolean
  Constant3 : Constant  OutDataTypeStr=boolean
  Data Type Conversion : DataTypeConversion  OutDataTypeStr=uint16  SaturateOnIntegerOverflow=off  RndMeth=Floor
  OR : Logic  Operator=OR  AllPortsSameDT=off  OutDataTypeStr=boolean
  Relational Operator : RelationalOperator  Operator=<  OutDataTypeStr=boolean  RndMeth=Simplest  InputSameDT=off
  Relational Operator1 : RelationalOperator  Operator=>  OutDataTypeStr=boolean  RndMeth=Simplest  InputSameDT=off
  Switch : Switch  Criteria=u2 > Threshold  SaturateOnIntegerOverflow=off  InputSameDT=off
  Switch1 : Switch  Criteria=u2 > Threshold  SaturateOnIntegerOverflow=off  InputSameDT=off
  Unit Delay : UnitDelay  SampleTime=-1  HasFrameUpgradeWarning=on
  WSS_FL_L1p_Calculation : Subsystem  TreatAsAtomicUnit=on
  m/s to Kmph : Gain  Gain=3.6
  WSS_FL_Valid_Flg : Outport
  WSS_FL_L1p : Outport  Port=2
  wires:
  m/s to Kmph/1 -> Data Type Conversion/1
  [WhlSpdFL_Phy_Kph] -> Relational Operator/1
  Constant/1 -> Relational Operator/2
  [WhlSpdFL_Phy_Kph] -> Relational Operator1/1
  Constant1/1 -> Relational Operator1/2
  Relational Operator/1 -> OR/1
  Relational Operator1/1 -> OR/2
  OR/1 -> [WhlSpdFL_Valid_Chk]  "WhlSpdFL_Valid_Chk"
  [WhlSpdFL_Valid_Chk] -> Switch/2
  Switch/1 -> WSS_FL_Valid_Flg/1  "WSS_FL_Valid_Flg"
  Constant2/1 -> Switch/1
  Constant3/1 -> Switch/3
  [WhlSpdFL_Valid_Chk] -> Switch1/2
  Switch1/1 -> Unit Delay/1, WSS_FL_L1p/1  "WSS_FL_L1p"
  WSS_FL_L1p_Calculation/1(WSS_FL_L1p) -> Switch1/3
  Unit Delay/1 -> [WSS_FL_L1p_Prev]  "WSS_FL_L1p_Prev"
  [WSS_FL_L1p_Prev] -> WSS_FL_L1p_Calculation/2(WSS_FL_L1p_Prev)
  [WhlSpdFL_Phy_Kph] -> WSS_FL_L1p_Calculation/1(WhlSpdFL_Phy_Kph)
  [WSS_FL_L1p_Prev] -> Switch1/1
  Alpha_WSS/1 -> WSS_FL_L1p_Calculation/3(Alpha)
  WhlSpdFL_m/s/1 -> m/s to Kmph/1
  Data Type Conversion/1 -> [WhlSpdFL_Phy_Kph]  "WhlSpdFR_Phy_Kph"

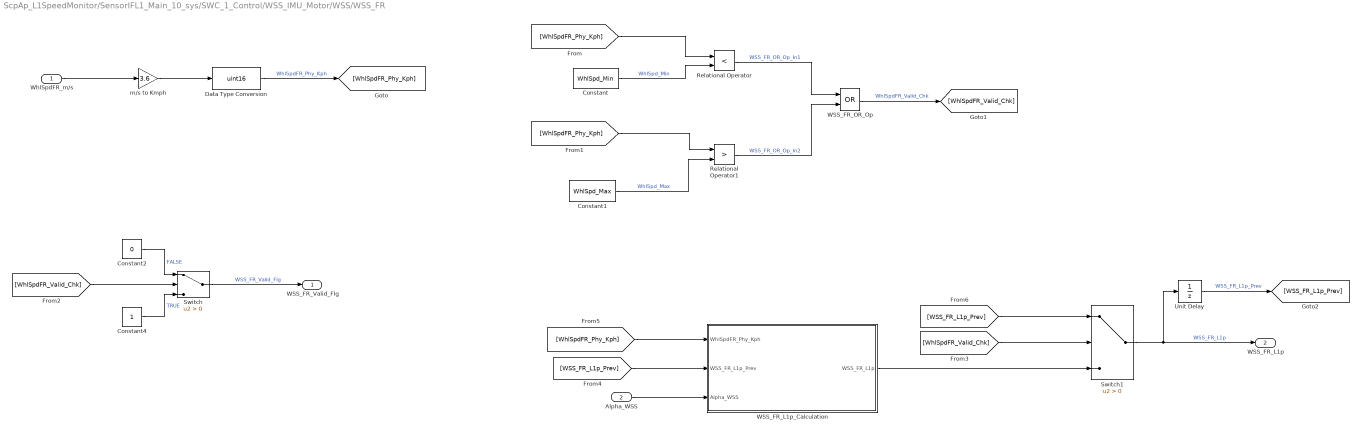
== system ScpAp_L1SpeedMonitor/SensorIFL1_Main_10_sys/SWC_1_Control/WSS_IMU_Motor/WSS/WSS_FR ==
  WhlSpdFR_m/s : Inport
  Alpha_WSS : Inport  Port=2
  Constant : Constant  Value=WhlSpd_Min
  Constant1 : Constant  Value=WhlSpd_Max
  Constant2 : Constant  Value=0  OutDataTypeStr=boolean
  Constant4 : Constant  OutDataTypeStr=boolean
  Data Type Conversion : DataTypeConversion  OutDataTypeStr=uint16  SaturateOnIntegerOverflow=off  RndMeth=Floor
  Relational Operator : RelationalOperator  Operator=<  OutDataTypeStr=boolean  RndMeth=Simplest  InputSameDT=off
  Relational Operator1 : RelationalOperator  Operator=>  OutDataTypeStr=boolean  RndMeth=Simplest  InputSameDT=off
  Switch : Switch  Criteria=u2 > Threshold  OutDataTypeStr=boolean  SaturateOnIntegerOverflow=off  InputSameDT=off
  Switch1 : Switch  Criteria=u2 > Threshold  SaturateOnIntegerOverflow=off  InputSameDT=off
  Unit Delay : UnitDelay  SampleTime=-1  HasFrameUpgradeWarning=on
  WSS_FR_L1p_Calculation : Subsystem  TreatAsAtomicUnit=on
  WSS_FR_OR_Op : Logic  Operator=OR  AllPortsSameDT=off  OutDataTypeStr=boolean
  m/s to Kmph : Gain  Gain=3.6
  WSS_FR_Valid_Flg : Outport  OutDataTypeStr=boolean
  WSS_FR_L1p : Outport  Port=2
  wires:
  m/s to Kmph/1 -> Data Type Conversion/1
  Relational Operator1/1 -> WSS_FR_OR_Op/2  "WSS_FR_OR_Op_In2"
  WSS_FR_OR_Op/1 -> [WhlSpdFR_Valid_Chk]  "WhlSpdFR_Valid_Chk"
  [WhlSpdFR_Valid_Chk] -> Switch/2
  Switch/1 -> WSS_FR_Valid_Flg/1  "WSS_FR_Valid_Flg"
  [WhlSpdFR_Valid_Chk] -> Switch1/2
  Switch1/1 -> Unit Delay/1, WSS_FR_L1p/1  "WSS_FR_L1p"
  WSS_FR_L1p_Calculation/1(WSS_FR_L1p) -> Switch1/3
  Unit Delay/1 -> [WSS_FR_L1p_Prev]  "WSS_FR_L1p_Prev"
  [WSS_FR_L1p_Prev] -> WSS_FR_L1p_Calculation/2(WSS_FR_L1p_Prev)
  [WhlSpdFR_Phy_Kph] -> WSS_FR_L1p_Calculation/1(WhlSpdFR_Phy_Kph)
  [WSS_FR_L1p_Prev] -> Switch1/1
  Alpha_WSS/1 -> WSS_FR_L1p_Calculation/3(Alpha_WSS)
  WhlSpdFR_m/s/1 -> m/s to Kmph/1
  Constant2/1 -> Switch/1  "FALSE"
  Constant4/1 -> Switch/3  "TRUE"
  Relational Operator/1 -> WSS_FR_OR_Op/1  "WSS_FR_OR_Op_In1"
  Constant/1 -> Relational Operator/2  "WhlSpd_Min"
  [WhlSpdFR_Phy_Kph] -> Relational Operator/1
  [WhlSpdFR_Phy_Kph] -> Relational Operator1/1
  Constant1/1 -> Relational Operator1/2  "WhlSpd_Max"
  Data Type Conversion/1 -> [WhlSpdFR_Phy_Kph]  "WhlSpdFR_Phy_Kph"

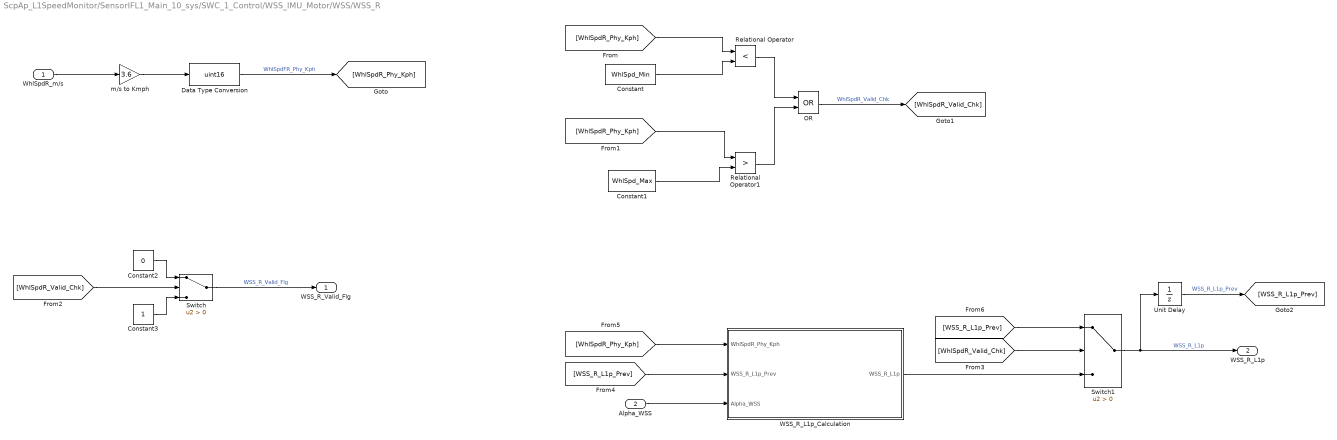
== system ScpAp_L1SpeedMonitor/SensorIFL1_Main_10_sys/SWC_1_Control/WSS_IMU_Motor/WSS/WSS_R ==
  WhlSpdR_m/s : Inport
  Alpha_WSS : Inport  Port=2
  Constant : Constant  Value=WhlSpd_Min
  Constant1 : Constant  Value=WhlSpd_Max
  Constant2 : Constant  Value=0  OutDataTypeStr=boolean
  Constant3 : Constant  OutDataTypeStr=boolean
  Data Type Conversion : DataTypeConversion  OutDataTypeStr=uint16  SaturateOnIntegerOverflow=off  RndMeth=Floor
  OR : Logic  Operator=OR  AllPortsSameDT=off  OutDataTypeStr=boolean
  Relational Operator : RelationalOperator  Operator=<  OutDataTypeStr=boolean  RndMeth=Simplest  InputSameDT=off
  Relational Operator1 : RelationalOperator  Operator=>  OutDataTypeStr=boolean  RndMeth=Simplest  InputSameDT=off
  Switch : Switch  Criteria=u2 > Threshold  SaturateOnIntegerOverflow=off  InputSameDT=off
  Switch1 : Switch  Criteria=u2 > Threshold  SaturateOnIntegerOverflow=off  InputSameDT=off
  Unit Delay : UnitDelay  SampleTime=-1  HasFrameUpgradeWarning=on
  WSS_R_L1p_Calculation : Subsystem  TreatAsAtomicUnit=on
  m/s to Kmph : Gain  Gain=3.6
  WSS_R_Valid_Flg : Outport
  WSS_R_L1p : Outport  Port=2
  wires:
  m/s to Kmph/1 -> Data Type Conversion/1
  [WhlSpdR_Phy_Kph] -> Relational Operator/1
  Constant/1 -> Relational Operator/2
  [WhlSpdR_Phy_Kph] -> Relational Operator1/1
  Constant1/1 -> Relational Operator1/2
  Relational Operator/1 -> OR/1
  Relational Operator1/1 -> OR/2
  OR/1 -> [WhlSpdR_Valid_Chk]  "WhlSpdR_Valid_Chk"
  [WhlSpdR_Valid_Chk] -> Switch/2
  Switch/1 -> WSS_R_Valid_Flg/1  "WSS_R_Valid_Flg"
  Constant2/1 -> Switch/1
  Constant3/1 -> Switch/3
  [WhlSpdR_Valid_Chk] -> Switch1/2
  Switch1/1 -> Unit Delay/1, WSS_R_L1p/1  "WSS_R_L1p"
  WSS_R_L1p_Calculation/1(WSS_R_L1p) -> Switch1/3
  Unit Delay/1 -> [WSS_R_L1p_Prev]  "WSS_R_L1p_Prev"
  [WSS_R_L1p_Prev] -> WSS_R_L1p_Calculation/2(WSS_R_L1p_Prev)
  [WhlSpdR_Phy_Kph] -> WSS_R_L1p_Calculation/1(WhlSpdR_Phy_Kph)
  [WSS_R_L1p_Prev] -> Switch1/1
  Alpha_WSS/1 -> WSS_R_L1p_Calculation/3(Alpha_WSS)
  WhlSpdR_m/s/1 -> m/s to Kmph/1
  Data Type Conversion/1 -> [WhlSpdR_Phy_Kph]  "WhlSpdFR_Phy_Kph"

== system ScpAp_L1SpeedMonitor/SensorIFL1_Main_10_sys/SWC_1_Control/WSS_IMU_Motor/WSS/WSS_FL/WSS_FL_L1p_Calculation ==
  WhlSpdFL_Phy_Kph : Inport
  WSS_FL_L1p_Prev : Inport  Port=2
  Alpha : Inport  Port=3
  Add : Sum
  Constant : Constant  OutDataTypeStr=uint16
  Product : Product  OutDataTypeStr=uint16
  Product1 : Product  OutDataTypeStr=uint16
  Subtract : Sum  Inputs=+-  OutDataTypeStr=uint16
  WSS_FL_L1p : Outport
  wires:
  WhlSpdFL_Phy_Kph/1 -> Product/1
  Alpha/1 -> [Alpha]
  [Alpha] -> Product/2
  [Alpha] -> Subtract/2
  Constant/1 -> Subtract/1
  Subtract/1 -> Product1/1
  WSS_FL_L1p_Prev/1 -> Product1/2
  Product/1 -> Add/1
  Product1/1 -> Add/2
  Add/1 -> WSS_FL_L1p/1  "WSS_FL_L1p"

== system ScpAp_L1SpeedMonitor/SensorIFL1_Main_10_sys/SWC_1_Control/WSS_IMU_Motor/WSS/WSS_FR/WSS_FR_L1p_Calculation ==
  WhlSpdFR_Phy_Kph : Inport
  WSS_FR_L1p_Prev : Inport  Port=2
  Alpha_WSS : Inport  Port=3
  Add : Sum
  Constant : Constant  OutDataTypeStr=uint16
  Product : Product  OutDataTypeStr=uint16
  Product1 : Product  OutDataTypeStr=uint16
  Subtract : Sum  Inputs=+-  OutDataTypeStr=uint16
  WSS_FR_L1p : Outport
  wires:
  WhlSpdFR_Phy_Kph/1 -> Product/1
  Alpha_WSS/1 -> [Alpha_WSS]
  [Alpha_WSS] -> Product/2
  [Alpha_WSS] -> Subtract/2
  Constant/1 -> Subtract/1
  Subtract/1 -> Product1/1
  WSS_FR_L1p_Prev/1 -> Product1/2
  Product/1 -> Add/1
  Product1/1 -> Add/2
  Add/1 -> WSS_FR_L1p/1  "WSS_FR_L1p"

== system ScpAp_L1SpeedMonitor/SensorIFL1_Main_10_sys/SWC_1_Control/WSS_IMU_Motor/WSS/WSS_R/WSS_R_L1p_Calculation ==
  WhlSpdR_Phy_Kph : Inport
  WSS_R_L1p_Prev : Inport  Port=2
  Alpha_WSS : Inport  Port=3
  Add : Sum
  Constant : Constant  OutDataTypeStr=uint16
  Product : Product  OutDataTypeStr=uint16
  Product1 : Product  OutDataTypeStr=uint16
  Subtract : Sum  Inputs=+-  OutDataTypeStr=uint16
  WSS_R_L1p : Outport
  wires:
  WhlSpdR_Phy_Kph/1 -> Product/1
  Alpha_WSS/1 -> [Alpha_WSS]
  [Alpha_WSS] -> Product/2
  [Alpha_WSS] -> Subtract/2
  Constant/1 -> Subtract/1
  Subtract/1 -> Product1/1
  WSS_R_L1p_Prev/1 -> Product1/2
  Product/1 -> Add/1
  Product1/1 -> Add/2
  Add/1 -> WSS_R_L1p/1  "WSS_R_L1p"
